simulink model "WholeSystem"  (R2023a)
settings: Solver=VariableStepAuto  StartTime=0.0  StopTime=10.0  RelTol=1e-3
settings Model: Creator=19591  LastModifiedBy=19591

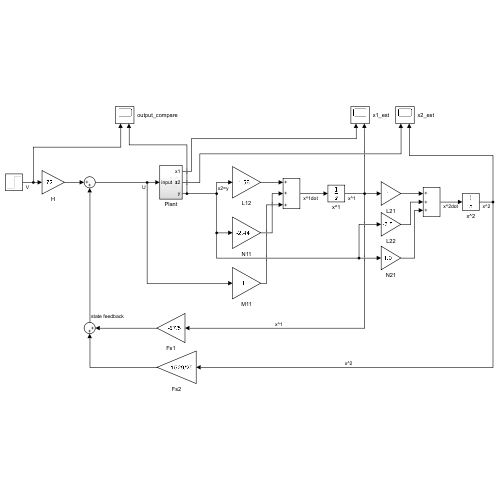
[thumbnail: Simulink's stored preview of the top-level diagram]
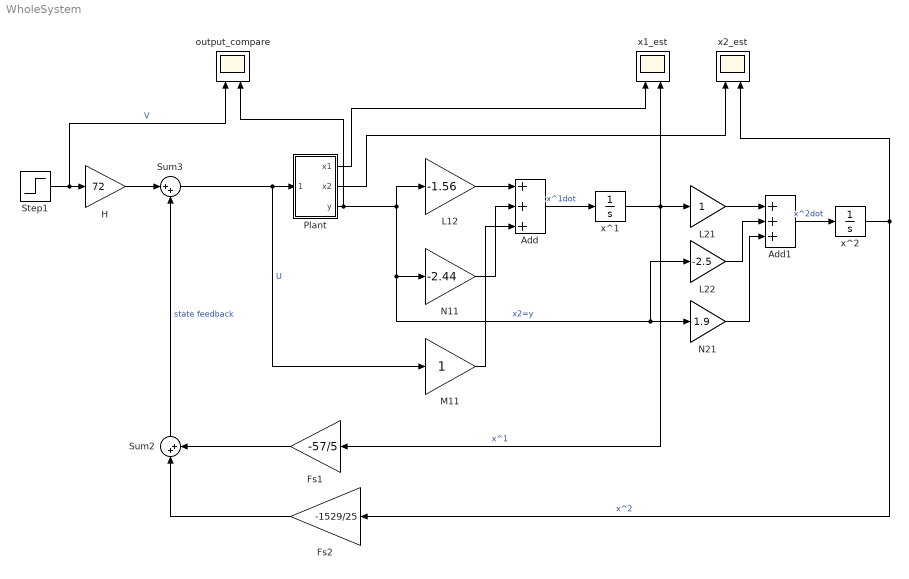
== system WholeSystem ==
  Add : Sum  Inputs=+++
  Add1 : Sum  Inputs=+++
  Fs1 : Gain  Gain=-57/5
  Fs2 : Gain  Gain=-1529/25
  H : Gain  Gain=72
  L12 : Gain  Gain=-1.56
  L21 : Gain
  L22 : Gain  Gain=-2.5
  M11 : Gain
  N11 : Gain  Gain=-2.44
  N21 : Gain  Gain=1.9
  Plant : Subsystem
  Step1 : Step  SampleTime=0
  Sum2 : Sum  Inputs=|++
  Sum3 : Sum  Inputs=|++
  output_compare : Scope  NumInputPorts=2
  x1_est : Scope  NumInputPorts=2
  x2_est : Scope  NumInputPorts=2
  x^1 : Integrator
  x^2 : Integrator
  wires:
  Plant/3(y) -> L12/1, L22/1, N21/1, N11/1, output_compare/2  "x2=y"
  L12/1 -> Add/1
  N11/1 -> Add/2
  M11/1 -> Add/3
  Add/1 -> x^1/1  "x^1dot"
  L22/1 -> Add1/2
  x^1/1 -> Fs1/1, L21/1, x1_est/2  "x^1"
  N21/1 -> Add1/3
  L21/1 -> Add1/1
  Add1/1 -> x^2/1  "x^2dot"
  x^2/1 -> Fs2/1, x2_est/2  "x^2"
  Plant/2(x2) -> x2_est/1
  Plant/1(x1) -> x1_est/1
  Step1/1 -> output_compare/1, H/1  "V"
  H/1 -> Sum3/1
  Sum3/1 -> M11/1, Plant/1(input)  "U"
  Sum2/1 -> Sum3/2  "state feedback"
  Fs1/1 -> Sum2/2
  Fs2/1 -> Sum2/1

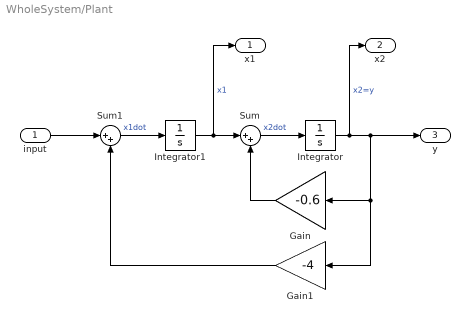
== system WholeSystem/Plant ==
  input : Inport
  Gain : Gain  Gain=-0.6
  Gain1 : Gain  Gain=-4
  Integrator : Integrator
  Integrator1 : Integrator
  Sum : Sum  Inputs=|++
  Sum1 : Sum  Inputs=|++
  x1 : Outport
  x2 : Outport  Port=2
  y : Outport  Port=3
  wires:
  input/1 -> Sum1/1
  Sum1/1 -> Integrator1/1  "x1dot"
  Gain1/1 -> Sum1/2
  Sum/1 -> Integrator/1  "x2dot"
  Integrator1/1 -> x1/1, Sum/1  "x1"
  Integrator/1 -> x2/1, y/1, Gain1/1, Gain/1  "x2=y"
  Gain/1 -> Sum/2
